simulink model "naibaoOSTBC_22_qpsk"  (R2018a)
settings: Solver=VariableStepAuto  StartTime=0.0  StopTime=10.0  RelTol=1e-3
model workspace (MAT data in the model file):
  FrameLength = 100
  SampleTime = 0.001
  maxNumBits = 100000000
  maxNumErrs = 1000
undefined symbols (not defined in the file): doppler
libraries: commchan3 x5, commmimo x2, commdigbbndpm3 x2, commrandsrc3 x1, commsink2 x1
settings Model: Creator=myste  LastModifiedBy=myste

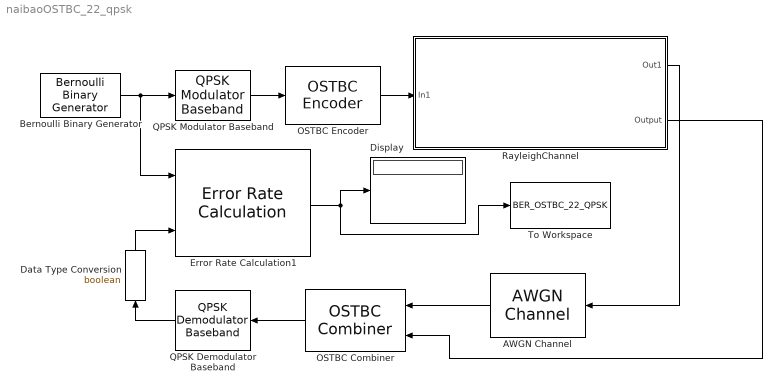
== system naibaoOSTBC_22_qpsk ==
  AWGN Channel : commchan3/AWGN Channel  InputProcessing=Columns as channels (frame based)  seed=67  noiseMode="Signal to noise ratio  (Eb/No)"  EbNodB=EbNo  EsNodB=10  SNRdB=10  bitsPerSym=2  Ps=2  Tsym=2*SampleTime  variance=1
  Bernoulli Binary Generator : commrandsrc3/Bernoulli Binary Generator  ProbabilityOfZero=0.5  SeedSource=Auto  Seed=1983  SampleTime=SampleTime  SamplesPerFrame=FrameLength  OutputDataType=boolean  SimulateUsing=Interpreted execution
  Data Type Conversion : DataTypeConversion  OutDataTypeStr=boolean
  Display : Display
  Error Rate Calculation1 : commsink2/Error Rate Calculation  N=0  st_delay=0  cp_mode=Entire frame  subframe=[]  PMode=Port  WsName=ErrorVec  RsMode2=off  stop=on  numErr=maxNumErrs  maxBits=maxNumBits
  OSTBC Combiner : commmimo/OSTBC Combiner  numTx=2  rate=3/4  numRx=2  roundingMode=Floor  overflowMode=Wrap  OvFlMode=off  OvFlModeLastStrValue=off  crossProductWordLen=32  crossProductFracLen=16  crossSumWordLen=32  crossSumFracLen=16  egyProductWordLen=32  egyProductFracLen=16  egySumWordLen=32  egySumFracLen=16  divisionWordLen=32  divisionFracLen=16  divisionDataTypeStr=Inherit: Same as accumulator  divisionLastDataTypeStr=Inherit: Same as accumulator
      settings: SourceProductName=Communications System Toolbox  SourceProductBaseCode=CM
  OSTBC Encoder : commmimo/OSTBC Encoder  numTx=2  rate=3/4  overflowMode=Wrap  OvFlMode=off  OvFlModeLastStrValue=off
      settings: SourceProductName=Communications System Toolbox  SourceProductBaseCode=CM
  QPSK Demodulator Baseband : commdigbbndpm3/QPSK Demodulator Baseband  OutType=Bit  DecType=Hard decision  VarSource=Dialog  Variance=1  Dec=Gray  Ph=0  outDtype1=Inherit via internal rule  outDtype2=Inherit via internal rule  derotateFactorWordLen=16  derotateFactorDataTypeStr=Inherit: Same word length as input  derotateFactorLastDataTypeStr=Inherit: Same word length as input
  QPSK Modulator Baseband : commdigbbndpm3/QPSK Modulator Baseband  InType=Bit  Enc=Gray  Ph=0  outDtype=double  outWordLen=16  outUDDataType=sfix(16)  outFracLenMode=Best precision  outFracLen=15  outDataTypeStr=double  outLastDataTypeStr=double
  RayleighChannel : Subsystem
  To Workspace : ToWorkspace  VariableName=BER_OSTBC_22_QPSK  SampleTime=-1
      settings: MaxDataPoints=1  Save2DSignal=2-D array (concatenate along first dimension)
  wires:
  Bernoulli Binary Generator/1 -> Error Rate Calculation1/1, QPSK Modulator Baseband/1
  QPSK Modulator Baseband/1 -> OSTBC Encoder/1
  OSTBC Encoder/1 -> RayleighChannel/1(In1)
  AWGN Channel/1 -> OSTBC Combiner/1
  RayleighChannel/1(Out1) -> AWGN Channel/1
  RayleighChannel/2(Output) -> OSTBC Combiner/2
  OSTBC Combiner/1 -> QPSK Demodulator Baseband/1
  Error Rate Calculation1/1 -> To Workspace/1, Display/1
  Data Type Conversion/1 -> Error Rate Calculation1/2
  QPSK Demodulator Baseband/1 -> Data Type Conversion/1

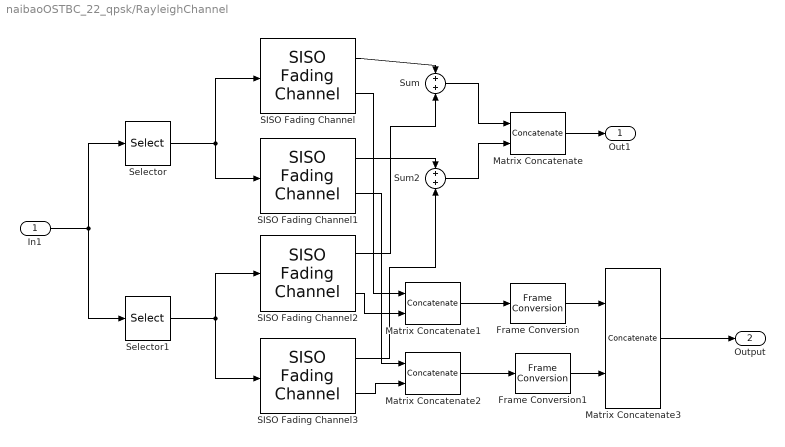
== system naibaoOSTBC_22_qpsk/RayleighChannel ==
  In1 : Inport
  Frame Conversion : FrameConversion  OutFrame=Sample-based
  Frame Conversion1 : FrameConversion  OutFrame=Sample-based
  Matrix Concatenate : Concatenate  Mode=Multidimensional array  ConcatenateDimension=2
  Matrix Concatenate1 : Concatenate  Mode=Multidimensional array  ConcatenateDimension=2
  Matrix Concatenate2 : Concatenate  Mode=Multidimensional array  ConcatenateDimension=2
  Matrix Concatenate3 : Concatenate  Mode=Multidimensional array  ConcatenateDimension=3
  SISO Fading Channel : commchan3/SISO Fading Channel  InheritSampleRate=on  SampleRate=1  PathDelays=0  AveragePathGains=0  NormalizePathGains=on  FadingDistribution=Rayleigh  KFactor=3  DirectPathDopplerShift=0  DirectPathInitialPhase=0  MaximumDopplerShift=3  DopplerSpectrum=doppler('Jakes')  ChannelInterpolationMethod=Polyphase  RandomStream=mt19937ar with seed  RandomNumGenerator=mt19937ar  Seed=123  PathGainsOutputPort=on  ChannelFilterDelayOutputPort=off  SimulateUsing=Interpreted execution  Visualization=Off  PathsForDopplerDisplay=1  SamplesToDisplay=25%
      settings: SourceProductName=Communications System Toolbox
  SISO Fading Channel1 : commchan3/SISO Fading Channel  InheritSampleRate=on  SampleRate=1  PathDelays=0  AveragePathGains=0  NormalizePathGains=on  FadingDistribution=Rayleigh  KFactor=3  DirectPathDopplerShift=0  DirectPathInitialPhase=0  MaximumDopplerShift=3  DopplerSpectrum=doppler('Jakes')  ChannelInterpolationMethod=Polyphase  RandomStream=mt19937ar with seed  RandomNumGenerator=mt19937ar  Seed=73  PathGainsOutputPort=on  ChannelFilterDelayOutputPort=off  SimulateUsing=Interpreted execution  Visualization=Off  PathsForDopplerDisplay=1  SamplesToDisplay=25%
      settings: SourceProductName=Communications System Toolbox
  SISO Fading Channel2 : commchan3/SISO Fading Channel  InheritSampleRate=on  SampleRate=1  PathDelays=0  AveragePathGains=0  NormalizePathGains=on  FadingDistribution=Rayleigh  KFactor=3  DirectPathDopplerShift=0  DirectPathInitialPhase=0  MaximumDopplerShift=3  DopplerSpectrum=doppler('Jakes')  ChannelInterpolationMethod=Polyphase  RandomStream=mt19937ar with seed  RandomNumGenerator=mt19937ar  Seed=88  PathGainsOutputPort=on  ChannelFilterDelayOutputPort=off  SimulateUsing=Interpreted execution  Visualization=Off  PathsForDopplerDisplay=1  SamplesToDisplay=25%
      settings: SourceProductName=Communications System Toolbox
  SISO Fading Channel3 : commchan3/SISO Fading Channel  InheritSampleRate=on  SampleRate=1  PathDelays=0  AveragePathGains=0  NormalizePathGains=on  FadingDistribution=Rayleigh  KFactor=3  DirectPathDopplerShift=0  DirectPathInitialPhase=0  MaximumDopplerShift=3  DopplerSpectrum=doppler('Jakes')  ChannelInterpolationMethod=Polyphase  RandomStream=mt19937ar with seed  RandomNumGenerator=mt19937ar  Seed=95  PathGainsOutputPort=on  ChannelFilterDelayOutputPort=off  SimulateUsing=Interpreted execution  Visualization=Off  PathsForDopplerDisplay=1  SamplesToDisplay=25%
      settings: SourceProductName=Communications System Toolbox
  Selector : Selector  NumberOfDimensions=2  InputPortWidth=3  IndexOptions=Select all,Index vector (dialog)  Indices=[1 3],1  OutputSizes=1,1
  Selector1 : Selector  NumberOfDimensions=2  InputPortWidth=3  IndexOptions=Select all,Index vector (dialog)  Indices=[1 3],2  OutputSizes=1,1
  Sum : Sum
  Sum2 : Sum
  Out1 : Outport
  Output : Outport  Port=2
  wires:
  In1/1 -> Selector1/1, Selector/1
  Selector/1 -> SISO Fading Channel/1, SISO Fading Channel1/1
  Selector1/1 -> SISO Fading Channel3/1, SISO Fading Channel2/1
  SISO Fading Channel/1 -> Sum/1
  SISO Fading Channel2/1 -> Sum/2
  SISO Fading Channel1/1 -> Sum2/1
  Sum/1 -> Matrix Concatenate/1
  Sum2/1 -> Matrix Concatenate/2
  SISO Fading Channel/2 -> Matrix Concatenate1/1
  SISO Fading Channel3/1 -> Sum2/2
  SISO Fading Channel2/2 -> Matrix Concatenate1/2
  SISO Fading Channel1/2 -> Matrix Concatenate2/1
  SISO Fading Channel3/2 -> Matrix Concatenate2/2
  Matrix Concatenate/1 -> Out1/1
  Matrix Concatenate1/1 -> Frame Conversion/1
  Matrix Concatenate2/1 -> Frame Conversion1/1
  Frame Conversion1/1 -> Matrix Concatenate3/2
  Frame Conversion/1 -> Matrix Concatenate3/1
  Matrix Concatenate3/1 -> Output/1
